simulink library "Power_Control_Axle2_FixedRatio"  (R2025a)
settings: Solver=VariableStepAuto  StartTime=0.0  StopTime=10.0  RelTol=1e-3
undefined symbols (not defined in the file): Control
Description:
  | Simscape Vehicle Templates Library
  | 
  | Copyright 2018-2025 The MathWorks, Inc.
settings Model: Creator=smiller  LastModifiedBy=smiller
settings ModelReferenceCC: EnableRefExpFcnMdlSchedulingChecks=on
settings RTWCC: GPUComputeCapability=3.5

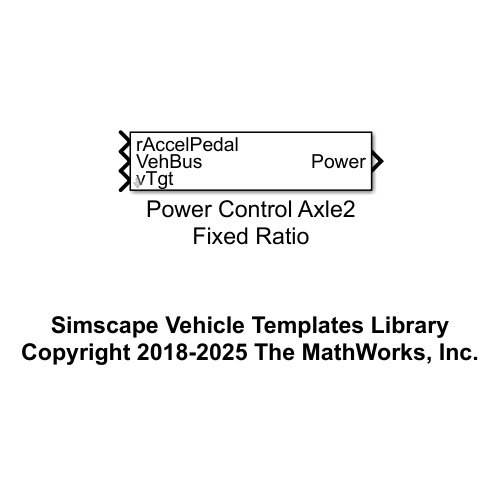
[thumbnail: Simulink's stored preview of the top-level diagram]
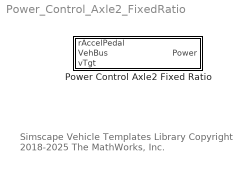
== system Power_Control_Axle2_FixedRatio ==
  note: Simscape Vehicle Templates Library
      | Copyright 2018-2025 The MathWorks, Inc.
  Power Control Axle2 Fixed Ratio : Subsystem  mask{trq_max=Control.Default.maxTrqRequest, trq_ratio_front=Control.Default.pcnt_torque_on_f, trq_rate_up=300, trq_rate_down=-5000}
      mask prompts: trq_max "Max Torque Request"; trq_ratio_front "Ratio of Torque on Front Wheels (0-1)"; trq_rate_up "Torque Rate Limit Up (N*m/s)"; trq_rate_down "Torque Rate Limit Down (N*m/s)"

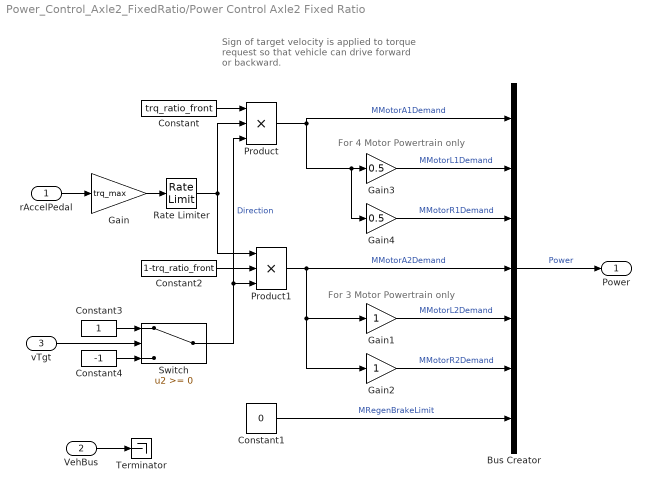
== system Power_Control_Axle2_FixedRatio/Power Control Axle2 Fixed Ratio ==
  note: Sign of target velocity is applied to torque request so that vehicle can drive forward or backward.
  note: For 3 Motor Powertrain only
  note: For 4 Motor Powertrain only
  rAccelPedal : Inport
  VehBus : Inport  Port=2
  vTgt : Inport  Port=3
  Bus Creator : BusCreator  Inputs=7
  Constant : Constant  Value=trq_ratio_front
  Constant1 : Constant  Value=0
  Constant2 : Constant  Value=1-trq_ratio_front
  Constant3 : Constant
  Constant4 : Constant  Value=-1
  Gain : Gain  Gain=trq_max
  Gain1 : Gain
  Gain2 : Gain
  Gain3 : Gain  Gain=0.5
  Gain4 : Gain  Gain=0.5
  Product : Product  Inputs=3
  Product1 : Product  Inputs=3
  Rate Limiter : RateLimiter  RisingSlewLimit=trq_rate_up  FallingSlewLimit=trq_rate_down  SampleTimeMode=inherited
  Switch : Switch  ZeroCross=off  SaturateOnIntegerOverflow=off  InputSameDT=off
  Terminator : Terminator
  Power : Outport  VectorParamsAs1DForOutWhenUnconnected=off
  wires:
  Constant4/1 -> Switch/3
  Constant3/1 -> Switch/1
  Switch/1 -> Product1/3, Product/3  "Direction"
  vTgt/1 -> Switch/2
  Gain4/1 -> Bus Creator/3  "MMotorR1Demand"
  Gain3/1 -> Bus Creator/2  "MMotorL1Demand"
  Gain2/1 -> Bus Creator/6  "MMotorR2Demand"
  Gain1/1 -> Bus Creator/5  "MMotorL2Demand"
  Constant2/1 -> Product1/2
  Constant/1 -> Product/1
  Rate Limiter/1 -> Product/2, Product1/1
  Constant1/1 -> Bus Creator/7  "MRegenBrakeLimit"
  VehBus/1 -> Terminator/1
  rAccelPedal/1 -> Gain/1
  Product/1 -> Gain3/1, Gain4/1, Bus Creator/1  "MMotorA1Demand"
  Gain/1 -> Rate Limiter/1
  Product1/1 -> Bus Creator/4, Gain1/1, Gain2/1  "MMotorA2Demand"
  Bus Creator/1 -> Power/1  "Power"
